simulink model "twotank"  (Simulink 9.2)
settings: Solver=VariableStepAuto  StartTime=0.0  StopTime=50  MaxStep=1e-3  RelTol=1e-3
settings Model: Creator=jinwooro  LastModifiedBy=jinwooro  NumberOfSteps=10000
settings DataIOCC: LimitDataPoints=off  SaveFormat=Dataset  SignalLoggingSaveFormat=Dataset
settings OptimizationCC: LifeSpan=auto
settings DebuggingCC: UnderspecifiedInitializationDetection=Simplified  MergeDetectMultiDrivingBlocksExec=error  FcnCallInpInsideContextMsg=error  StateNameClashWarn=none  SFUnexpectedBacktrackingDiag=error  SFNoUnconditionalDefaultTransitionDiag=error  SFExecutionAtInitializationDiag=warning
settings HardwareCC: ProdBitPerPointer=64  ProdBitPerSizeT=64  ProdBitPerPtrDiffT=64  ProdLargestAtomicFloat=Float  ProdIntDivRoundTo=Zero  ProdEndianess=LittleEndian  ProdWordSize=64  ProdHWDeviceType=Intel->x86-64 (Windows64)
settings ModelReferenceCC: PropagateSignalLabelsOutOfModel=on
settings SFSimCC: SimUseLocalCustomCode=on
settings RTWCC: RTWUseLocalCustomCode=on
settings CodeAppCC: StateflowObjectComments=off
settings GRTTargetCC: TargetLangStandard=C99 (ISO)  GeneratePreprocessorConditionals=Use local settings  CombineOutputUpdateFcns=on  GRTInterface=off
settings ConfigComp: CovMetricSettings=dwe  CovHtmlReporting=off  CovSaveCumulativeToWorkspaceVar=off  CovSaveSingleToWorkspaceVar=off  CovExternalEMLEnable=on

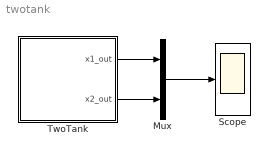
== system twotank ==
  Mux : Mux  Inputs=2
  Scope : Scope
  TwoTank : Stateflow chart  TreatAsAtomicUnit=on
  wires:
  Mux/1 -> Scope/1
  TwoTank/1(x1_out) -> Mux/1
  TwoTank/2(x2_out) -> Mux/2

== stateflow chart TwoTank ==
  settings: updateMethod=CONTINUOUS
  state Loc1
    du:
    x1_dot = 3.5 - power(x1 - x2 + 15, 0.5);
    x2_dot = power( x1 - x2 + 15, 0.5) - power(x2, 0.5);
    x1_out = x1;
    x2_out = x2;
  state Loc2
    du:
    x1_dot = 3.5 - power(x1,0.5);
    x2_dot = power(x1,0.5) - power(x2,0.5);
    x1_out = x1;
    x2_out = x2;
  (default) -> Loc1 : {
      | x1 = 50;
      | x2 = 10;
      | }
  Loc1 -> Loc2 : [x2 <= 15]
  Loc2 -> Loc1 : [x2 > 15]
  data: x1 local double; x2 local double; x1_out output double; x2_out output double
  data x1 settings: updateMethod=SF_CONTINUOUS_TIME_DATA
  data x2 settings: updateMethod=SF_CONTINUOUS_TIME_DATA
